simulink model "FullStateFeedbackSimulation"  (R2018b)
settings: Solver=VariableStepAuto  StartTime=0.0  StopTime=10  RelTol=1e-3
values from neighbouring files (symbols this model uses):
  K = place(linsyspendulum.A, linsyspendulum.B, poles)    [LinearizePendulumRCSPlant.m]
settings Model: Creator=mendicantbias  LastModifiedBy=mendicantbias
settings ModelReferenceCC: ModelReferenceMinAlgLoopOccurrences=on

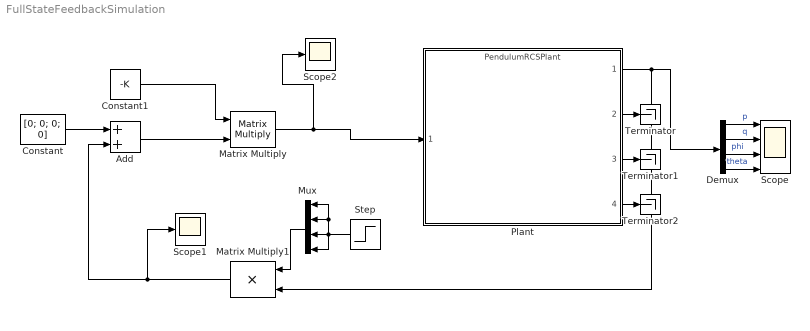
== system FullStateFeedbackSimulation ==
  Add : Sum
  Constant : Constant  Value=[0; 0; 0; 0]
  Constant1 : Constant  Value=-K
  Demux : Demux
  Matrix Multiply : Product  Multiplication=Matrix(*)
  Matrix Multiply1 : Product
  Mux : Mux
  Plant : ModelReference  ModelNameDialog=PendulumRCSPlant  SimulationMode=Normal  ModelReferenceVersion=1.182
  Scope : Scope  NumInputPorts=4
  Scope1 : Scope
  Scope2 : Scope
  Step : Step  Time=5  SampleTime=0
  Terminator : Terminator
  Terminator1 : Terminator
  Terminator2 : Terminator
  wires:
  Constant/1 -> Add/1
  Matrix Multiply1/1 -> Scope1/1, Add/2
  Demux/4 -> Scope/4  "theta"
  Demux/3 -> Scope/3  "phi"
  Demux/2 -> Scope/2  "q"
  Demux/1 -> Scope/1  "p"
  Mux/1 -> Matrix Multiply1/1
  Step/1 -> Mux/3, Mux/2, Mux/1, Mux/4
  Plant/1 -> Matrix Multiply1/2, Demux/1
  Matrix Multiply/1 -> Scope2/1, Plant/1
  Add/1 -> Matrix Multiply/2
  Constant1/1 -> Matrix Multiply/1
  Plant/2 -> Terminator/1
  Plant/3 -> Terminator1/1
  Plant/4 -> Terminator2/1
